simulink model "carsim1"  (R2017b)
settings: Solver=VariableStepAuto  StartTime=0.0  StopTime=50  RelTol=1e-3
libraries: Solver_SF x1
settings Model: Creator=lancer  LastModifiedBy=lancer

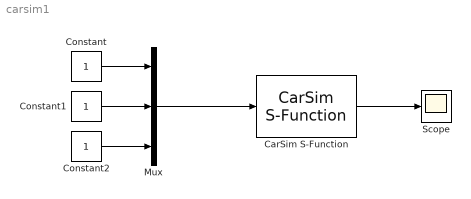
== system carsim1 ==
  CarSim S-Function : Solver_SF/CarSim S-Function  Priority=1  VehicleCode=i_i  SIMFILE=simfile
  Constant : Constant
  Constant1 : Constant
  Constant2 : Constant
  Mux : Mux  Inputs=3
  Scope : Scope
  wires:
  Mux/1 -> CarSim S-Function/1
  Constant/1 -> Mux/1
  Constant1/1 -> Mux/2
  Constant2/1 -> Mux/3
  CarSim S-Function/1 -> Scope/1
